simulink model "sys_model"  (R2021a)
settings: Solver=FixedStepAuto  StartTime=0.0  StopTime=10  MaxStep=0.001  RelTol=1e-3
settings Model: Creator=Admin  LastModifiedBy=Rushikesh
settings SolverCC: AlgebraicLoopSolver=TrustRegion
settings DebuggingCC: SFMachineParentedDataDiag=warning

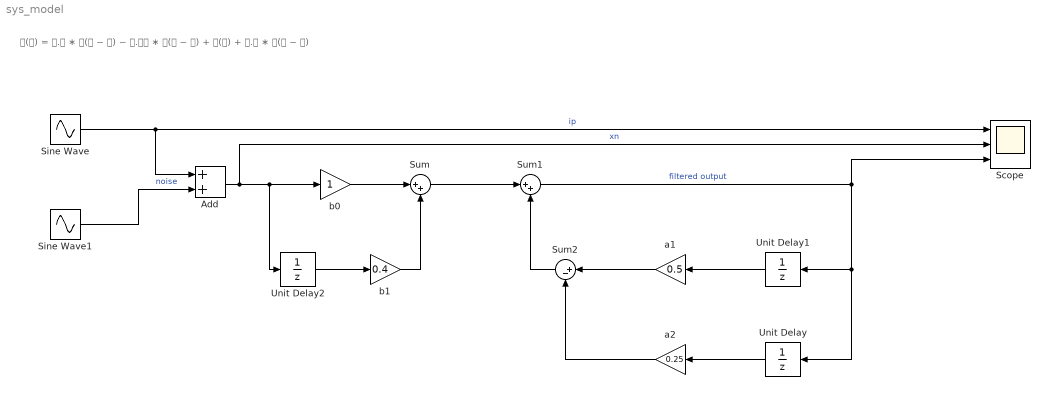
== system sys_model ==
  note: 𝐲(𝐧) = 𝟎.𝟓 ∗ 𝐲(𝐧 − 𝟏) − 𝟎.𝟐𝟓 ∗ 𝐲(𝐧 − 𝟐) + 𝐱(𝐧) + 𝟎.𝟒 ∗ 𝐱(𝐧 − 𝟏)
  Add : Sum
  Scope : Scope  NumInputPorts=3
  Sine Wave : Sin  Frequency=5  SampleTime=0
  Sine Wave1 : Sin  Frequency=1000  SampleTime=0
  Sum : Sum  Inputs=|++
  Sum1 : Sum  Inputs=|++
  Sum2 : Sum  Inputs=|+-
  Unit Delay : UnitDelay  SampleTime=-1  HasFrameUpgradeWarning=on
  Unit Delay1 : UnitDelay  SampleTime=-1  HasFrameUpgradeWarning=on
  Unit Delay2 : UnitDelay  SampleTime=-1  HasFrameUpgradeWarning=on
  a1 : Gain  Gain=0.5
  a2 : Gain  Gain=0.25
  b0 : Gain
  b1 : Gain  Gain=0.4
  wires:
  Add/1 -> Scope/2, Unit Delay2/1, b0/1  "xn"
  b0/1 -> Sum/1
  Unit Delay2/1 -> b1/1
  b1/1 -> Sum/2
  Sum/1 -> Sum1/1
  Sum2/1 -> Sum1/2
  Sum1/1 -> Scope/3, Unit Delay/1, Unit Delay1/1  "filtered output"
  Unit Delay/1 -> a2/1
  Unit Delay1/1 -> a1/1
  a1/1 -> Sum2/1
  a2/1 -> Sum2/2
  Sine Wave/1 -> Add/1, Scope/1  "ip"
  Sine Wave1/1 -> Add/2  "noise"
